simulink library "pwrsysTransf"  (R2016a)
settings: Solver=VariableStepAuto  SolverMode=SingleTasking  StartTime=0.0  StopTime=10.0  RelTol=1e-3
undefined symbols (not defined in the file or in its folder): fn
undefined symbols (not defined in the file): Ts_control
libraries: powerlib_meascontrol x32, pwrsysBasic x12, peTransforms x12, pwrsysTransf x12, pwrsysAMA x4, cstblocks x2
settings Model: Creator=daniemot  LastModifiedBy=ericfa
settings DebuggingCC: SFUnexpectedBacktrackingDiag=error  SFNoUnconditionalDefaultTransitionDiag=error
settings GRTTargetCC: TargetLangStandard=C99 (ISO)  GeneratePreprocessorConditionals=Use local settings
settings ConfigComp: CovMetricSettings=dwe  CovHtmlReporting=off  CovSaveCumulativeToWorkspaceVar=off  CovSaveSingleToWorkspaceVar=off  CovExternalEMLEnable=on

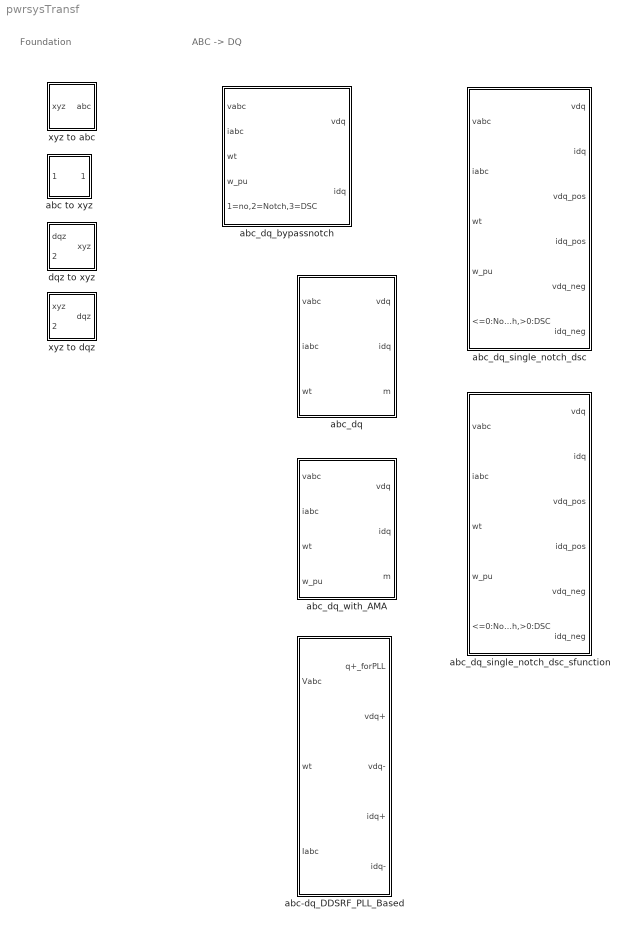
== system pwrsysTransf ==
  note: ABC -> DQ
  note: Foundation
  abc to xyz : Subsystem  mask(Clarke transformation){typeTransf=Amplitude-invariant}
      mask prompts: typeTransf "Type of transformation"
      mask init:
      | switch typeTransf
      |     case 1
      |         a = 1/3;
      |         b = 1/sqrt(3);
      |         c = sqrt(2)/3;
      |     case 2
      |         a = 1/sqrt(6);
      |         b = 1/sqrt(2);
      |         c = 1/sqrt(3);
      | end
      mask TypeOptions typeTransf: Amplitude-invariant | Power-invariant
  abc-dq_DDSRF_PLL_Based : Subsystem  mask(abc -> dq based on DDSRF PLL){Ts=Ts_control, fc=fn/2^0.5}
      mask prompts: Ts "Sampling time [s]"; fc "Cutout freq. low pass [Hz]"
      mask help:
      | abc -> dq transducer based on the Decoupled Double Synchronous Reference Frame PLL for Power Converters Control from Rodriguez 2007.
      | The PLL is not implemented, but an output with eq is available for using in a PLL
  abc_dq : Subsystem  mask(abc->dq with Matlab){Ts=0.001, fn=100, fcutoutv=1000, fcutouti=1000, zeta=0.707}
      mask prompts: Ts "Sampling time [s]"; fn "Notch frequency [Hz]"; fcutoutv "Cutout freq. low-pass for vdq meas. [Hz]"; fcutouti "Cutout freq. low-pass for idq meas. [Hz]"; zeta "Zeta for notch filters"
  abc_dq_bypassnotch : Subsystem  mask(abc->dq with Matlab){Ts=0.001, fn=100, fcutoutv=1000, fcutouti=1000, zeta=0.707}
      mask prompts: Ts "Sampling time [s]"; fn "Notch frequency [Hz]"; fcutoutv "Cutout freq. low-pass for vdq meas. [Hz]"; fcutouti "Cutout freq. low-pass for idq meas. [Hz]"; zeta "Zeta for notch filters"
      mask help:
      | To be done
      |
      | Max buffer size for DSC 500 samples
  abc_dq_single_notch_dsc : Subsystem  mask(abc->dq with Matlab){Ts=0.001, fn=100, zeta=0.707}
      mask prompts: Ts "Sampling time [s]"; fn "Notch frequency [Hz]"; zeta "Zeta for notch filters"
      mask help:
      | To be done
      |
      | Max buffer size for DSC 500 samples
  abc_dq_single_notch_dsc_sfunction : Subsystem  mask(abc->dq with Matlab){Ts=0.001, fn=100, zeta=0.707}
      mask prompts: Ts "Sampling time [s]"; fn "Notch frequency [Hz]"; zeta "Zeta for notch filters"
      mask help:
      | To be done
      |
      | Max buffer size for DSC 500 samples
  abc_dq_with_AMA : Subsystem  mask(abc->dq with Matlab){Ts=0.001, fn=100, fmin=0, fmax=0, fcutoutv=1000, fcutouti=1000}
      mask prompts: Ts "Sampling time [s]"; fn "Rated grid frequency [Hz]"; fmin "Min. acceptable grid freq [Hz]"; fmax "Max. acceptable grid freq [Hz]"; fcutoutv "Cutout freq. low-pass for vdq meas. [Hz]"; fcutouti "Cutout freq. low-pass for idq meas. [Hz]"
  dqz to xyz : Subsystem  mask(Inverse Park transformation){}
  xyz to abc : Subsystem  mask(Inverse Clarke transformation){typeTransf=Amplitude-invariant}
      mask prompts: typeTransf "Type of transformation"
      mask init:
      | switch typeTransf
      |     case 1
      |         a = 1;
      |         b = sqrt(3)/2;
      |         c = 1/2;
      |         d = 1/sqrt(2);
      |     case 2
      |         a = sqrt(2/3);
      |         b = 1/sqrt(2);
      |         c = 1/sqrt(6);
      |         d = 1/sqrt(3);
      | end
      mask TypeOptions typeTransf: Amplitude-invariant | Power-invariant
  xyz to dqz : Subsystem  mask(Inverse Park transformation){}

== system pwrsysTransf/abc to xyz ==
  note: Clark Transform
  abc : Inport
  Demux : Demux  Outputs=3
  Gain : Gain  Gain=c
  Gain1 : Gain  Gain=a
  Gain2 : Gain  Gain=b
  Gain4 : Gain  Gain=2
  Mux : Mux  Inputs=3
  Sum1 : Sum  Inputs=+-
  Sum2 : Sum  Inputs=+++
  Sum3 : Sum  Inputs=+--
  xyz : Outport
  wires:
  abc/1 -> Demux/1
  Demux/1 -> Sum2/1, Gain4/1  "a"
  Gain/1 -> Mux/3  "z"
  Gain2/1 -> Mux/2  "y"
  Gain1/1 -> Mux/1  "x"
  Mux/1 -> xyz/1
  Gain4/1 -> Sum3/1
  Demux/2 -> Sum2/2, Sum1/1, Sum3/2  "b"
  Demux/3 -> Sum2/3, Sum1/2, Sum3/3  "c"
  Sum3/1 -> Gain1/1  "B"
  Sum1/1 -> Gain2/1
  Sum2/1 -> Gain/1

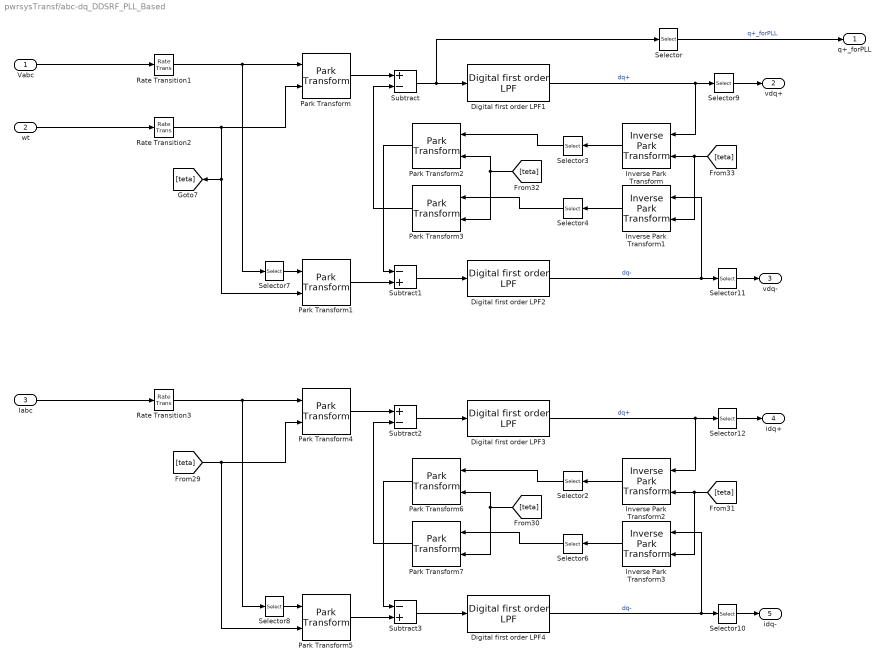
== system pwrsysTransf/abc-dq_DDSRF_PLL_Based ==
  Vabc : Inport
  wt : Inport  Port=2
  Iabc : Inport  Port=3
  Digital first order LPF{1..4} (4 alike) : pwrsysBasic/Digital first order LPF  Ts=Ts  fcutout=fc
  Inverse Park Transform{,1..3} (4 alike) : peTransforms/Inverse Park Transform  AxisAlignment=Q-axis  PowerInvariant=off
  Park Transform{,1..7} (8 alike) : peTransforms/Park Transform  AxisAlignment=Q-axis  PowerInvariant=off
  Rate Transition1 : RateTransition  OutPortSampleTime=Ts
  Rate Transition2 : RateTransition  OutPortSampleTime=Ts
  Rate Transition3 : RateTransition  OutPortSampleTime=Ts
  Selector : Selector  InputPortWidth=3  IndexOptions=Index vector (dialog)  Indices=2  OutputSizes=1
  Selector{9..12} (4 alike) : Selector  InputPortWidth=3  IndexOptions=Index vector (dialog)  Indices=[1 2]  OutputSizes=1
  Selector{2..4,6..8} (6 alike) : Selector  InputPortWidth=3  IndexOptions=Index vector (dialog)  Indices=[1 3 2]  OutputSizes=1
  Subtract : Sum  Inputs=+-
  Subtract1 : Sum  Inputs=-+
  Subtract2 : Sum  Inputs=+-
  Subtract3 : Sum  Inputs=-+
  q+_forPLL : Outport
  vdq+ : Outport  Port=2
  vdq- : Outport  Port=3
  idq+ : Outport  Port=4
  idq- : Outport  Port=5
  wires:
  Selector/1 -> q+_forPLL/1  "q+_forPLL"
  [teta] -> Inverse Park Transform2/2, Inverse Park Transform3/2
  Rate Transition3/1 -> Selector8/1, Park Transform4/1
  Selector11/1 -> vdq-/1
  Rate Transition1/1 -> Selector7/1, Park Transform/1
  Digital first order LPF4/1 -> Inverse Park Transform3/1, Selector10/1  "dq-"
  Inverse Park Transform3/1 -> Selector6/1
  Rate Transition2/1 -> [teta], Park Transform1/2, Park Transform/2
  Selector4/1 -> Park Transform3/1
  Iabc/1 -> Rate Transition3/1
  [teta] -> Park Transform6/2, Park Transform7/2
  Subtract2/1 -> Digital first order LPF3/1
  Park Transform1/1 -> Subtract1/2
  Selector6/1 -> Park Transform7/1
  Selector8/1 -> Park Transform5/1
  Park Transform7/1 -> Subtract2/2
  Digital first order LPF2/1 -> Selector11/1, Inverse Park Transform1/1  "dq-"
  Selector9/1 -> vdq+/1
  Inverse Park Transform1/1 -> Selector4/1
  Inverse Park Transform2/1 -> Selector2/1
  [teta] -> Park Transform2/2, Park Transform3/2
  Selector10/1 -> idq-/1
  Park Transform2/1 -> Subtract1/1
  Selector2/1 -> Park Transform6/1
  Park Transform5/1 -> Subtract3/2
  Subtract3/1 -> Digital first order LPF4/1
  Subtract1/1 -> Digital first order LPF2/1
  Park Transform/1 -> Subtract/1
  Digital first order LPF3/1 -> Inverse Park Transform2/1, Selector12/1  "dq+"
  Selector12/1 -> idq+/1
  Selector3/1 -> Park Transform2/1
  wt/1 -> Rate Transition2/1
  Park Transform6/1 -> Subtract3/1
  [teta] -> Park Transform5/2, Park Transform4/2
  Park Transform4/1 -> Subtract2/1
  Subtract/1 -> Digital first order LPF1/1, Selector/1
  [teta] -> Inverse Park Transform/2, Inverse Park Transform1/2
  Digital first order LPF1/1 -> Selector9/1, Inverse Park Transform/1  "dq+"
  Vabc/1 -> Rate Transition1/1
  Selector7/1 -> Park Transform1/1
  Inverse Park Transform/1 -> Selector3/1
  Park Transform3/1 -> Subtract/2

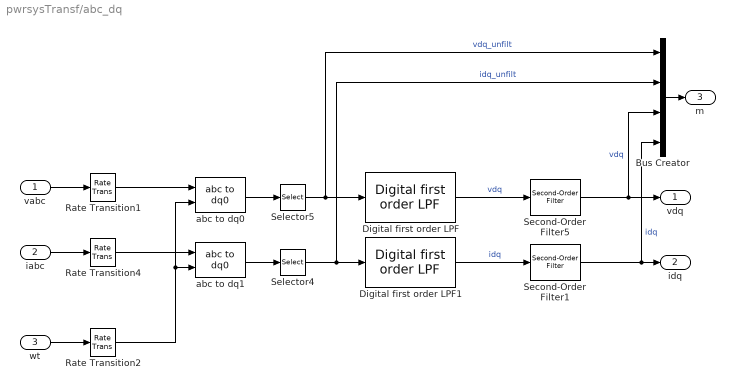
== system pwrsysTransf/abc_dq ==
  vabc : Inport
  iabc : Inport  Port=2
  wt : Inport  Port=3
  Bus Creator : BusCreator  Inputs=4
  Digital first order LPF : pwrsysBasic/Digital first order LPF  Ts=Ts  fcutout=fcutoutv
  Digital first order LPF1 : pwrsysBasic/Digital first order LPF  Ts=Ts  fcutout=fcutouti
  Rate Transition1 : RateTransition  OutPortSampleTime=Ts
  Rate Transition2 : RateTransition  OutPortSampleTime=Ts
  Rate Transition4 : RateTransition  OutPortSampleTime=Ts
  Second-Order Filter1 : powerlib_meascontrol/Filters/Second-Order Filter  FilterType=Bandstop (Notch)  Fo=fn  Zeta=zeta  Ts=Ts  Initialize=off  Vac_Init="[0,  0,  60]"  Vdc_Init=0  PlotResponse=off  FreqRange=[0, 1000, 0.1]
  Second-Order Filter5 : powerlib_meascontrol/Filters/Second-Order Filter  FilterType=Bandstop (Notch)  Fo=fn  Zeta=zeta  Ts=Ts  Initialize=off  Vac_Init="[0,  0,  60]"  Vdc_Init=0  PlotResponse=off  FreqRange=[0, 1000, 0.1]
  Selector4 : Selector  InputPortWidth=3  IndexOptions=Index vector (dialog)  Indices=[1 2]  OutputSizes=1
  Selector5 : Selector  InputPortWidth=3  IndexOptions=Index vector (dialog)  Indices=[1 2]  OutputSizes=1
  abc to dq0 : powerlib_meascontrol/Transformations/abc to dq0  Alignment=90 degrees behind phase A axis
  abc to dq1 : powerlib_meascontrol/Transformations/abc to dq0  Alignment=90 degrees behind phase A axis
  vdq : Outport
  idq : Outport  Port=2
  m : Outport  Port=3
  wires:
  abc to dq1/1 -> Selector4/1
  Selector5/1 -> Digital first order LPF/1, Bus Creator/1  "vdq_unfilt"
  Rate Transition1/1 -> abc to dq0/1
  Rate Transition2/1 -> abc to dq1/2, abc to dq0/2
  Selector4/1 -> Bus Creator/2, Digital first order LPF1/1  "idq_unfilt"
  Rate Transition4/1 -> abc to dq1/1
  abc to dq0/1 -> Selector5/1
  Bus Creator/1 -> m/1
  Second-Order Filter5/1 -> vdq/1, Bus Creator/3  "vdq"
  wt/1 -> Rate Transition2/1
  vabc/1 -> Rate Transition1/1
  iabc/1 -> Rate Transition4/1
  Digital first order LPF1/1 -> Second-Order Filter1/1  "idq"
  Digital first order LPF/1 -> Second-Order Filter5/1  "vdq"
  Second-Order Filter1/1 -> Bus Creator/4, idq/1  "idq"

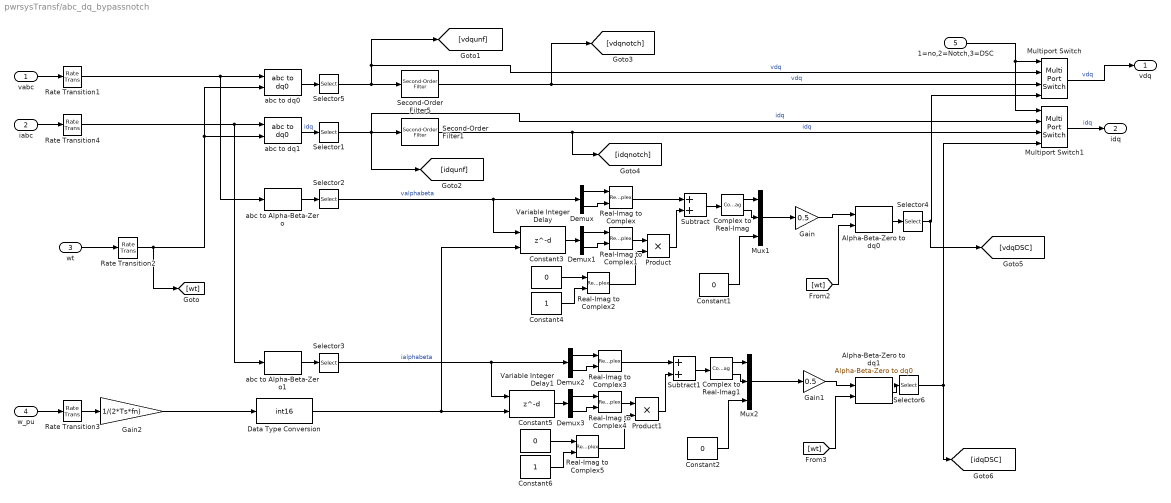
== system pwrsysTransf/abc_dq_bypassnotch ==
  vabc : Inport
  iabc : Inport  Port=2
  wt : Inport  Port=3
  w_pu : Inport  Port=4
  1=no,2=Notch,3=DSC : Inport  Port=5
  Alpha-Beta-Zero to dq0 : powerlib_meascontrol/Transformations/Alpha-Beta-Zero to dq0  Alignment=90 degrees behind phase A axis
  Alpha-Beta-Zero to dq1 : powerlib_meascontrol/Transformations/Alpha-Beta-Zero to dq0  Alignment=90 degrees behind phase A axis
  Complex to Real-Imag : ComplexToRealImag
  Complex to Real-Imag1 : ComplexToRealImag
  Constant{1..3,5} (4 alike) : Constant  Value=0
  Constant4 : Constant
  Constant6 : Constant
  Data Type Conversion : DataTypeConversion  OutDataTypeStr=int16  RndMeth=Round  SaturateOnIntegerOverflow=on
  Demux{,1..3} (4 alike) : Demux  Outputs=2
  Gain : Gain  Gain=0.5
  Gain1 : Gain  Gain=0.5
  Gain2 : Gain  Gain=1/(2*Ts*fn)
  Multiport Switch : MultiPortSwitch
  Multiport Switch1 : MultiPortSwitch
  Mux1 : Mux  Inputs=[1 1 1]
  Mux2 : Mux  Inputs=[1 1 1]
  Product : Product
  Product1 : Product
  Rate Transition1 : RateTransition  OutPortSampleTime=Ts
  Rate Transition2 : RateTransition  OutPortSampleTime=Ts
  Rate Transition3 : RateTransition  X0=1  OutPortSampleTime=Ts
  Rate Transition4 : RateTransition  OutPortSampleTime=Ts
  Real-Imag to Complex{,1..5} (6 alike) : RealImagToComplex
  Second-Order Filter1 : powerlib_meascontrol/Filters/Second-Order Filter  FilterType=Bandstop (Notch)  Fo=fn  Zeta=zeta  Ts=Ts  Initialize=off  Vac_Init="[0,  0,  60]"  Vdc_Init=0  PlotResponse=off  FreqRange=[0, 1000, 0.1]
  Second-Order Filter5 : powerlib_meascontrol/Filters/Second-Order Filter  FilterType=Bandstop (Notch)  Fo=fn  Zeta=zeta  Ts=Ts  Initialize=off  Vac_Init="[0,  0,  60]"  Vdc_Init=0  PlotResponse=off  FreqRange=[0, 1000, 0.1]
  Selector{1..6} (6 alike) : Selector  InputPortWidth=3  IndexOptions=Index vector (dialog)  Indices=[1 2]  OutputSizes=1
  Subtract : Sum
  Subtract1 : Sum
  Variable Integer Delay : Delay  DelayLengthSource=Input port  DelayLength=200  DelayLengthUpperLimit=500  SampleTime=Ts
      settings: InputPortMap=u0,p1
  Variable Integer Delay1 : Delay  DelayLengthSource=Input port  DelayLength=200  DelayLengthUpperLimit=500  SampleTime=Ts
      settings: InputPortMap=u0,p1
  abc to Alpha-Beta-Zero : powerlib_meascontrol/Transformations/abc to Alpha-Beta-Zero
  abc to Alpha-Beta-Zero1 : powerlib_meascontrol/Transformations/abc to Alpha-Beta-Zero
  abc to dq0 : powerlib_meascontrol/Transformations/abc to dq0  Alignment=90 degrees behind phase A axis
  abc to dq1 : powerlib_meascontrol/Transformations/abc to dq0  Alignment=90 degrees behind phase A axis
  vdq : Outport
  idq : Outport  Port=2
  wires:
  Rate Transition2/1 -> [wt], abc to dq1/2, abc to dq0/2
  wt/1 -> Rate Transition2/1
  abc to dq1/1 -> Selector1/1  "idq"
  Selector5/1 -> Second-Order Filter5/1, [vdqunf], Multiport Switch/2  "vdq"
  Second-Order Filter5/1 -> [vdqnotch], Multiport Switch/3  "vdq"
  Second-Order Filter1/1 -> [idqnotch], Multiport Switch1/3  "idq"
  abc to dq0/1 -> Selector5/1
  Selector1/1 -> [idqunf], Second-Order Filter1/1, Multiport Switch1/2  "idq"
  abc to Alpha-Beta-Zero/1 -> Selector2/1
  abc to Alpha-Beta-Zero1/1 -> Selector3/1
  Gain2/1 -> Data Type Conversion/1
  [wt] -> Alpha-Beta-Zero to dq0/2
  Alpha-Beta-Zero to dq0/1 -> Selector4/1
  Selector4/1 -> [vdqDSC], Multiport Switch/4
  Selector6/1 -> [idqDSC], Multiport Switch1/4
  [wt] -> Alpha-Beta-Zero to dq1/2
  Selector3/1 -> Demux2/1, Variable Integer Delay1/1  "ialphabeta"
  Alpha-Beta-Zero to dq1/1 -> Selector6/1
  Gain/1 -> Alpha-Beta-Zero to dq0/1
  Gain1/1 -> Alpha-Beta-Zero to dq1/1
  Variable Integer Delay/1 -> Demux1/1
  Constant1/1 -> Mux1/3
  Complex to Real-Imag/2 -> Mux1/2
  Constant4/1 -> Real-Imag to Complex2/2
  Complex to Real-Imag/1 -> Mux1/1
  Subtract/1 -> Complex to Real-Imag/1
  Real-Imag to Complex/1 -> Subtract/1
  Demux1/2 -> Real-Imag to Complex1/2
  Real-Imag to Complex1/1 -> Product/1
  Product/1 -> Subtract/2
  Real-Imag to Complex2/1 -> Product/2
  Constant3/1 -> Real-Imag to Complex2/1
  Demux1/1 -> Real-Imag to Complex1/1
  Demux/2 -> Real-Imag to Complex/2
  Demux/1 -> Real-Imag to Complex/1
  Selector2/1 -> Demux/1, Variable Integer Delay/1  "valphabeta"
  Mux1/1 -> Gain/1
  Mux2/1 -> Gain1/1
  Demux2/1 -> Real-Imag to Complex3/1
  Constant5/1 -> Real-Imag to Complex5/1
  Real-Imag to Complex5/1 -> Product1/2
  Demux3/1 -> Real-Imag to Complex4/1
  Product1/1 -> Subtract1/2
  Demux2/2 -> Real-Imag to Complex3/2
  Demux3/2 -> Real-Imag to Complex4/2
  Real-Imag to Complex3/1 -> Subtract1/1
  Constant6/1 -> Real-Imag to Complex5/2
  Real-Imag to Complex4/1 -> Product1/1
  Complex to Real-Imag1/1 -> Mux2/1
  Constant2/1 -> Mux2/3
  Complex to Real-Imag1/2 -> Mux2/2
  Variable Integer Delay1/1 -> Demux3/1
  Subtract1/1 -> Complex to Real-Imag1/1
  Rate Transition1/1 -> abc to Alpha-Beta-Zero/1, abc to dq0/1
  Rate Transition4/1 -> abc to Alpha-Beta-Zero1/1, abc to dq1/1
  w_pu/1 -> Rate Transition3/1
  Rate Transition3/1 -> Gain2/1
  vabc/1 -> Rate Transition1/1
  iabc/1 -> Rate Transition4/1
  Data Type Conversion/1 -> Variable Integer Delay1/2, Variable Integer Delay/2
  Multiport Switch/1 -> vdq/1  "vdq"
  Multiport Switch1/1 -> idq/1  "idq"
  1=no,2=Notch,3=DSC/1 -> Multiport Switch1/1, Multiport Switch/1

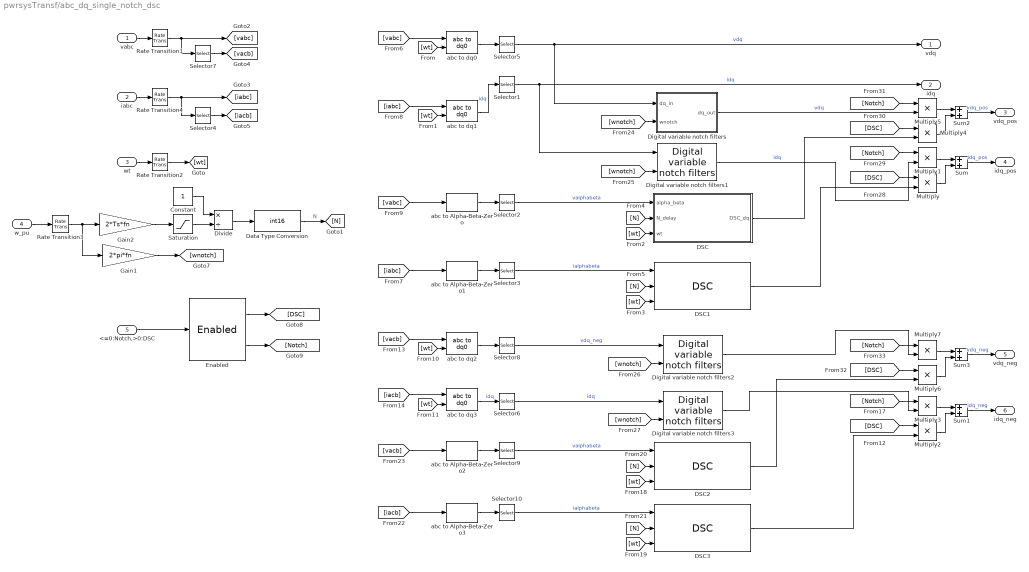
== system pwrsysTransf/abc_dq_single_notch_dsc ==
  vabc : Inport
  iabc : Inport  Port=2
  wt : Inport  Port=3
  w_pu : Inport  Port=4
  <=0:Notch,>0:DSC : Inport  Port=5
  Constant : Constant
  DSC : Subsystem
  DSC1 : pwrsysTransf/abc_dq_single_notch_dsc/DSC
  DSC2 : pwrsysTransf/abc_dq_single_notch_dsc/DSC
  DSC3 : pwrsysTransf/abc_dq_single_notch_dsc/DSC
  Data Type Conversion : DataTypeConversion  OutDataTypeStr=int16  RndMeth=Round  SaturateOnIntegerOverflow=on
  Digital variable notch filters : Subsystem
  Digital variable notch filters1 : pwrsysTransf/abc_dq_single_notch_dsc/Digital variable notch filters
  Digital variable notch filters2 : pwrsysTransf/abc_dq_single_notch_dsc/Digital variable notch filters
  Digital variable notch filters3 : pwrsysTransf/abc_dq_single_notch_dsc/Digital variable notch filters
  Divide : Product  Inputs=*/
  Enabled : pwrsysBasic/Enabled
  Gain1 : Gain  Gain=2*pi*fn
  Gain2 : Gain  Gain=2*Ts*fn
  Multiply{,1..7} (8 alike) : Product
  Rate Transition1 : RateTransition  OutPortSampleTime=Ts
  Rate Transition2 : RateTransition  OutPortSampleTime=Ts
  Rate Transition3 : RateTransition  X0=1  OutPortSampleTime=Ts
  Rate Transition4 : RateTransition  OutPortSampleTime=Ts
  Saturation : Saturate  UpperLimit=inf  LowerLimit=0.000001
  Selector{1..3,5..6,8..10} (8 alike) : Selector  InputPortWidth=3  IndexOptions=Index vector (dialog)  Indices=[1 2]  OutputSizes=1
  Selector4 : Selector  InputPortWidth=3  IndexOptions=Index vector (dialog)  Indices=[1 3 2]  OutputSizes=1
  Selector7 : Selector  InputPortWidth=3  IndexOptions=Index vector (dialog)  Indices=[1 3 2]  OutputSizes=1
  Sum{,1..3} (4 alike) : Sum
  abc to Alpha-Beta-Zero{,1..3} (4 alike) : powerlib_meascontrol/Transformations/abc to Alpha-Beta-Zero
  abc to dq{0..3} (4 alike) : powerlib_meascontrol/Transformations/abc to dq0  Alignment=90 degrees behind phase A axis
  vdq : Outport
  idq : Outport  Port=2
  vdq_pos : Outport  Port=3
  idq_pos : Outport  Port=4
  vdq_neg : Outport  Port=5
  idq_neg : Outport  Port=6
  wires:
  wt/1 -> Rate Transition2/1
  abc to dq1/1 -> Selector1/1  "idq"
  Selector5/1 -> Digital variable notch filters/1(dq_in), vdq/1  "vdq"
  abc to dq0/1 -> Selector5/1
  Selector1/1 -> Digital variable notch filters1/1, idq/1  "idq"
  abc to Alpha-Beta-Zero/1 -> Selector2/1
  abc to Alpha-Beta-Zero1/1 -> Selector3/1
  DSC/1(DSC_dq) -> Multiply4/2
  Selector3/1 -> DSC1/1  "ialphabeta"
  [vabc] -> abc to dq0/1
  [iabc] -> abc to dq1/1
  vabc/1 -> Rate Transition1/1
  iabc/1 -> Rate Transition4/1
  Selector2/1 -> DSC/1(alpha_beta)  "valphabeta"
  Digital variable notch filters/1(dq_out) -> Multiply5/2  "vdq"
  Digital variable notch filters1/1 -> Multiply1/2  "idq"
  DSC1/1 -> Multiply/2
  Sum2/1 -> vdq_pos/1  "vdq_pos"
  Sum/1 -> idq_pos/1  "idq_pos"
  Rate Transition2/1 -> [wt]
  [wt] -> abc to dq0/2
  [wt] -> abc to dq1/2
  [wt] -> DSC/3(wt)
  [wt] -> DSC1/3
  [N] -> DSC/2(N_delay)
  [N] -> DSC1/2
  Data Type Conversion/1 -> [N]  "N"
  Rate Transition1/1 -> Selector7/1, [vabc]
  Selector7/1 -> [vacb]
  Rate Transition4/1 -> Selector4/1, [iabc]
  Selector4/1 -> [iacb]
  [vabc] -> abc to Alpha-Beta-Zero/1
  [iabc] -> abc to Alpha-Beta-Zero1/1
  [wt] -> abc to dq3/2
  abc to dq2/1 -> Selector8/1
  Selector8/1 -> Digital variable notch filters2/1  "vdq_neg"
  [vacb] -> abc to dq2/1
  [wt] -> abc to dq2/2
  abc to dq3/1 -> Selector6/1  "idq"
  [iacb] -> abc to dq3/1
  Sum3/1 -> vdq_neg/1  "vdq_neg"
  Sum1/1 -> idq_neg/1  "idq_neg"
  Digital variable notch filters2/1 -> Multiply7/2
  Selector6/1 -> Digital variable notch filters3/1  "idq"
  Digital variable notch filters3/1 -> Multiply3/2
  abc to Alpha-Beta-Zero3/1 -> Selector10/1
  Selector10/1 -> DSC3/1  "ialphabeta"
  abc to Alpha-Beta-Zero2/1 -> Selector9/1
  [iacb] -> abc to Alpha-Beta-Zero3/1
  [wt] -> DSC2/3
  [vacb] -> abc to Alpha-Beta-Zero2/1
  DSC2/1 -> Multiply6/2
  Selector9/1 -> DSC2/1  "valphabeta"
  [N] -> DSC3/2
  [N] -> DSC2/2
  DSC3/1 -> Multiply2/2
  [wt] -> DSC3/3
  Gain2/1 -> Saturation/1
  Saturation/1 -> Divide/2
  Constant/1 -> Divide/1
  Rate Transition3/1 -> Gain1/1, Gain2/1
  Divide/1 -> Data Type Conversion/1
  w_pu/1 -> Rate Transition3/1
  Gain1/1 -> [wnotch]
  [wnotch] -> Digital variable notch filters/2(wnotch)
  [wnotch] -> Digital variable notch filters1/2
  [wnotch] -> Digital variable notch filters2/2
  [wnotch] -> Digital variable notch filters3/2
  <=0:Notch,>0:DSC/1 -> Enabled/1
  Enabled/1 -> [DSC]
  Enabled/2 -> [Notch]
  [DSC] -> Multiply/1
  [Notch] -> Multiply1/1
  Multiply1/1 -> Sum/1
  Multiply/1 -> Sum/2
  [Notch] -> Multiply3/1
  [DSC] -> Multiply2/1
  Multiply3/1 -> Sum1/1
  Multiply2/1 -> Sum1/2
  [Notch] -> Multiply5/1
  Multiply4/1 -> Sum2/2
  [DSC] -> Multiply4/1
  Multiply5/1 -> Sum2/1
  [Notch] -> Multiply7/1
  Multiply6/1 -> Sum3/2
  [DSC] -> Multiply6/1
  Multiply7/1 -> Sum3/1

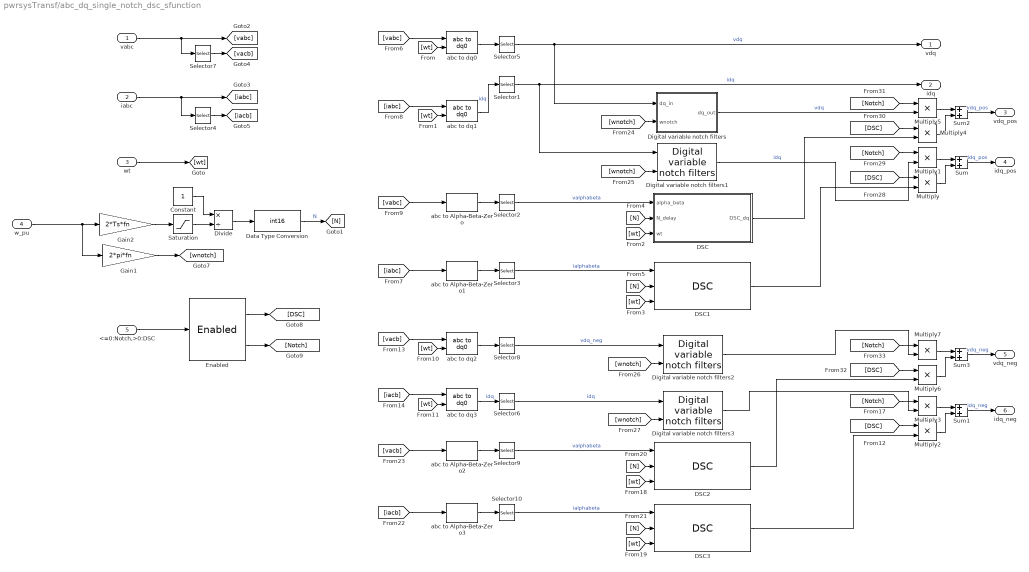
== system pwrsysTransf/abc_dq_single_notch_dsc_sfunction ==
  vabc : Inport
  iabc : Inport  Port=2
  wt : Inport  Port=3
  w_pu : Inport  Port=4
  <=0:Notch,>0:DSC : Inport  Port=5
  Constant : Constant
  DSC : Subsystem
  DSC1 : pwrsysTransf/abc_dq_single_notch_dsc/DSC
  DSC2 : pwrsysTransf/abc_dq_single_notch_dsc/DSC
  DSC3 : pwrsysTransf/abc_dq_single_notch_dsc/DSC
  Data Type Conversion : DataTypeConversion  OutDataTypeStr=int16  RndMeth=Round  SaturateOnIntegerOverflow=on
  Digital variable notch filters : Subsystem
  Digital variable notch filters1 : pwrsysTransf/abc_dq_single_notch_dsc_sfunction/Digital variable notch filters
  Digital variable notch filters2 : pwrsysTransf/abc_dq_single_notch_dsc_sfunction/Digital variable notch filters
  Digital variable notch filters3 : pwrsysTransf/abc_dq_single_notch_dsc_sfunction/Digital variable notch filters
  Divide : Product  Inputs=*/
  Enabled : pwrsysBasic/Enabled
  Gain1 : Gain  Gain=2*pi*fn
  Gain2 : Gain  Gain=2*Ts*fn
  Multiply{,1..7} (8 alike) : Product
  Saturation : Saturate  UpperLimit=inf  LowerLimit=0.000001
  Selector{1..3,5..6,8..10} (8 alike) : Selector  InputPortWidth=3  IndexOptions=Index vector (dialog)  Indices=[1 2]  OutputSizes=1
  Selector4 : Selector  InputPortWidth=3  IndexOptions=Index vector (dialog)  Indices=[1 3 2]  OutputSizes=1
  Selector7 : Selector  InputPortWidth=3  IndexOptions=Index vector (dialog)  Indices=[1 3 2]  OutputSizes=1
  Sum{,1..3} (4 alike) : Sum
  abc to Alpha-Beta-Zero{,1..3} (4 alike) : powerlib_meascontrol/Transformations/abc to Alpha-Beta-Zero
  abc to dq{0..3} (4 alike) : powerlib_meascontrol/Transformations/abc to dq0  Alignment=90 degrees behind phase A axis
  vdq : Outport
  idq : Outport  Port=2
  vdq_pos : Outport  Port=3
  idq_pos : Outport  Port=4
  vdq_neg : Outport  Port=5
  idq_neg : Outport  Port=6
  wires:
  Multiply7/1 -> Sum3/1
  [DSC] -> Multiply6/1
  Multiply6/1 -> Sum3/2
  [Notch] -> Multiply7/1
  Multiply5/1 -> Sum2/1
  [DSC] -> Multiply4/1
  Multiply4/1 -> Sum2/2
  [Notch] -> Multiply5/1
  Multiply2/1 -> Sum1/2
  Multiply3/1 -> Sum1/1
  [DSC] -> Multiply2/1
  [Notch] -> Multiply3/1
  Multiply/1 -> Sum/2
  Multiply1/1 -> Sum/1
  [Notch] -> Multiply1/1
  [DSC] -> Multiply/1
  Enabled/2 -> [Notch]
  Enabled/1 -> [DSC]
  <=0:Notch,>0:DSC/1 -> Enabled/1
  [wnotch] -> Digital variable notch filters3/2
  [wnotch] -> Digital variable notch filters2/2
  [wnotch] -> Digital variable notch filters1/2
  [wnotch] -> Digital variable notch filters/2(wnotch)
  Gain1/1 -> [wnotch]
  Divide/1 -> Data Type Conversion/1
  w_pu/1 -> Gain2/1, Gain1/1
  Constant/1 -> Divide/1
  Saturation/1 -> Divide/2
  Gain2/1 -> Saturation/1
  [wt] -> DSC3/3
  DSC3/1 -> Multiply2/2
  [N] -> DSC2/2
  [N] -> DSC3/2
  Selector9/1 -> DSC2/1  "valphabeta"
  DSC2/1 -> Multiply6/2
  [vacb] -> abc to Alpha-Beta-Zero2/1
  [wt] -> DSC2/3
  [iacb] -> abc to Alpha-Beta-Zero3/1
  abc to Alpha-Beta-Zero2/1 -> Selector9/1
  Selector10/1 -> DSC3/1  "ialphabeta"
  abc to Alpha-Beta-Zero3/1 -> Selector10/1
  Digital variable notch filters3/1 -> Multiply3/2
  Selector6/1 -> Digital variable notch filters3/1  "idq"
  Digital variable notch filters2/1 -> Multiply7/2
  Sum1/1 -> idq_neg/1  "idq_neg"
  Sum3/1 -> vdq_neg/1  "vdq_neg"
  [iacb] -> abc to dq3/1
  abc to dq3/1 -> Selector6/1  "idq"
  [wt] -> abc to dq2/2
  [vacb] -> abc to dq2/1
  Selector8/1 -> Digital variable notch filters2/1  "vdq_neg"
  abc to dq2/1 -> Selector8/1
  [wt] -> abc to dq3/2
  [iabc] -> abc to Alpha-Beta-Zero1/1
  [vabc] -> abc to Alpha-Beta-Zero/1
  Selector4/1 -> [iacb]
  iabc/1 -> [iabc], Selector4/1
  Selector7/1 -> [vacb]
  vabc/1 -> [vabc], Selector7/1
  Data Type Conversion/1 -> [N]  "N"
  [N] -> DSC1/2
  [N] -> DSC/2(N_delay)
  [wt] -> DSC1/3
  [wt] -> DSC/3(wt)
  [wt] -> abc to dq1/2
  [wt] -> abc to dq0/2
  wt/1 -> [wt]
  Sum/1 -> idq_pos/1  "idq_pos"
  Sum2/1 -> vdq_pos/1  "vdq_pos"
  DSC1/1 -> Multiply/2
  Digital variable notch filters1/1 -> Multiply1/2  "idq"
  Digital variable notch filters/1(dq_out) -> Multiply5/2  "vdq"
  Selector2/1 -> DSC/1(alpha_beta)  "valphabeta"
  [iabc] -> abc to dq1/1
  [vabc] -> abc to dq0/1
  Selector3/1 -> DSC1/1  "ialphabeta"
  DSC/1(DSC_dq) -> Multiply4/2
  abc to Alpha-Beta-Zero1/1 -> Selector3/1
  abc to Alpha-Beta-Zero/1 -> Selector2/1
  Selector1/1 -> Digital variable notch filters1/1, idq/1  "idq"
  abc to dq0/1 -> Selector5/1
  Selector5/1 -> vdq/1, Digital variable notch filters/1(dq_in)  "vdq"
  abc to dq1/1 -> Selector1/1  "idq"

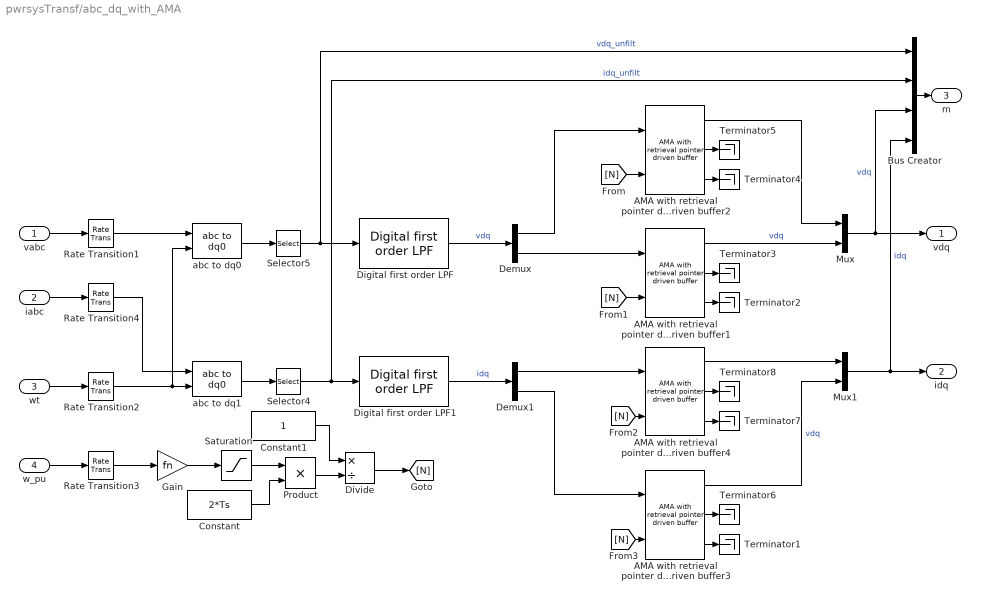
== system pwrsysTransf/abc_dq_with_AMA ==
  vabc : Inport
  iabc : Inport  Port=2
  wt : Inport  Port=3
  w_pu : Inport  Port=4
  AMA with retrieval pointer driven buffer{1..4} (4 alike) : pwrsysAMA/AMA with retrieval pointer driven buffer  NbSize=1/(2*fmin*Ts)  Ts=Ts
  Bus Creator : BusCreator  Inputs=4
  Constant : Constant  Value=2*Ts
  Constant1 : Constant
  Demux : Demux  Outputs=2
  Demux1 : Demux  Outputs=2
  Digital first order LPF : pwrsysBasic/Digital first order LPF  Ts=Ts  fcutout=fcutoutv
  Digital first order LPF1 : pwrsysBasic/Digital first order LPF  Ts=Ts  fcutout=fcutouti
  Divide : Product  Inputs=*/
  Gain : Gain  Gain=fn
  Mux : Mux  Inputs=2
  Mux1 : Mux  Inputs=2
  Product : Product
  Rate Transition1 : RateTransition  OutPortSampleTime=Ts
  Rate Transition2 : RateTransition  OutPortSampleTime=Ts
  Rate Transition3 : RateTransition  X0=1  OutPortSampleTime=Ts
  Rate Transition4 : RateTransition  OutPortSampleTime=Ts
  Saturation : Saturate  UpperLimit=fmax  LowerLimit=fmin
  Selector4 : Selector  InputPortWidth=3  IndexOptions=Index vector (dialog)  Indices=[1 2]  OutputSizes=1
  Selector5 : Selector  InputPortWidth=3  IndexOptions=Index vector (dialog)  Indices=[1 2]  OutputSizes=1
  Terminator{1..8} (8 alike) : Terminator
  abc to dq0 : powerlib_meascontrol/Transformations/abc to dq0  Alignment=90 degrees behind phase A axis
  abc to dq1 : powerlib_meascontrol/Transformations/abc to dq0  Alignment=90 degrees behind phase A axis
  vdq : Outport
  idq : Outport  Port=2
  m : Outport  Port=3
  wires:
  Digital first order LPF/1 -> Demux/1  "vdq"
  abc to dq1/1 -> Selector4/1
  Mux1/1 -> Bus Creator/4, idq/1  "idq"
  Selector5/1 -> Digital first order LPF/1, Bus Creator/1  "vdq_unfilt"
  Rate Transition1/1 -> abc to dq0/1
  Rate Transition2/1 -> abc to dq0/2, abc to dq1/2
  Selector4/1 -> Bus Creator/2, Digital first order LPF1/1  "idq_unfilt"
  Rate Transition4/1 -> abc to dq1/1
  abc to dq0/1 -> Selector5/1
  Bus Creator/1 -> m/1
  Mux/1 -> Bus Creator/3, vdq/1  "vdq"
  wt/1 -> Rate Transition2/1
  vabc/1 -> Rate Transition1/1
  iabc/1 -> Rate Transition4/1
  AMA with retrieval pointer driven buffer1/3 -> Terminator2/1
  AMA with retrieval pointer driven buffer1/2 -> Terminator3/1
  w_pu/1 -> Rate Transition3/1
  Rate Transition3/1 -> Gain/1
  Gain/1 -> Saturation/1
  Saturation/1 -> Product/1
  Constant/1 -> Product/2
  Product/1 -> Divide/2
  Constant1/1 -> Divide/1
  Divide/1 -> [N]
  Demux/1 -> AMA with retrieval pointer driven buffer2/1
  Demux/2 -> AMA with retrieval pointer driven buffer1/1
  AMA with retrieval pointer driven buffer2/3 -> Terminator4/1
  AMA with retrieval pointer driven buffer2/2 -> Terminator5/1
  AMA with retrieval pointer driven buffer2/1 -> Mux/1
  AMA with retrieval pointer driven buffer1/1 -> Mux/2  "vdq"
  AMA with retrieval pointer driven buffer3/1 -> Mux1/2  "vdq"
  AMA with retrieval pointer driven buffer4/2 -> Terminator8/1
  Demux1/1 -> AMA with retrieval pointer driven buffer4/1
  Demux1/2 -> AMA with retrieval pointer driven buffer3/1
  AMA with retrieval pointer driven buffer4/3 -> Terminator7/1
  AMA with retrieval pointer driven buffer3/3 -> Terminator1/1
  AMA with retrieval pointer driven buffer4/1 -> Mux1/1
  AMA with retrieval pointer driven buffer3/2 -> Terminator6/1
  Digital first order LPF1/1 -> Demux1/1  "idq"
  [N] -> AMA with retrieval pointer driven buffer2/2
  [N] -> AMA with retrieval pointer driven buffer1/2
  [N] -> AMA with retrieval pointer driven buffer4/2
  [N] -> AMA with retrieval pointer driven buffer3/2

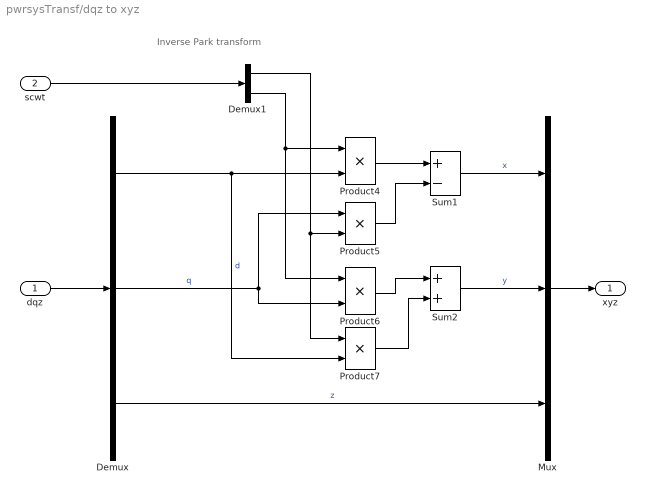
== system pwrsysTransf/dqz to xyz ==
  note: Inverse Park transform
  dqz : Inport
  scwt : Inport  Port=2
  Demux : Demux  Outputs=3
  Demux1 : Demux  Outputs=2
  Mux : Mux  Inputs=3
  Product{4..7} (4 alike) : Product
  Sum1 : Sum  Inputs=+-
  Sum2 : Sum
  xyz : Outport
  wires:
  dqz/1 -> Demux/1
  Demux/1 -> Product7/2, Product4/2  "d"
  Demux1/2 -> Product4/1, Product6/1
  Product5/1 -> Sum1/2
  Product4/1 -> Sum1/1
  Demux1/1 -> Product7/1, Product5/2
  Demux/2 -> Product6/2, Product5/1  "q"
  scwt/1 -> Demux1/1
  Product6/1 -> Sum2/1
  Product7/1 -> Sum2/2
  Mux/1 -> xyz/1
  Demux/3 -> Mux/3  "z"
  Sum2/1 -> Mux/2  "y"
  Sum1/1 -> Mux/1  "x"

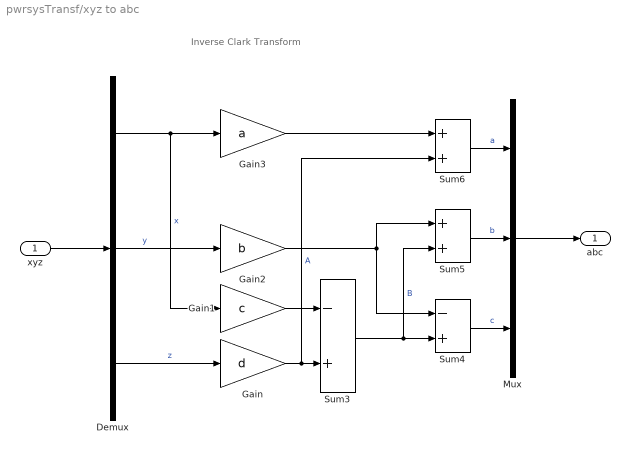
== system pwrsysTransf/xyz to abc ==
  note: Inverse Clark Transform
  xyz : Inport
  Demux : Demux  Outputs=3
  Gain : Gain  Gain=d
  Gain1 : Gain  Gain=c
  Gain2 : Gain  Gain=b
  Gain3 : Gain  Gain=a
  Mux : Mux  Inputs=3
  Sum3 : Sum  Inputs=-+
  Sum4 : Sum  Inputs=-+
  Sum5 : Sum
  Sum6 : Sum
  abc : Outport
  wires:
  xyz/1 -> Demux/1
  Demux/2 -> Gain2/1  "y"
  Demux/1 -> Gain3/1, Gain1/1  "x"
  Demux/3 -> Gain/1  "z"
  Gain1/1 -> Sum3/1
  Gain/1 -> Sum6/2, Sum3/2  "A"
  Gain2/1 -> Sum5/1, Sum4/1
  Sum3/1 -> Sum5/2, Sum4/2  "B"
  Sum4/1 -> Mux/3  "c"
  Sum5/1 -> Mux/2  "b"
  Sum6/1 -> Mux/1  "a"
  Gain3/1 -> Sum6/1
  Mux/1 -> abc/1

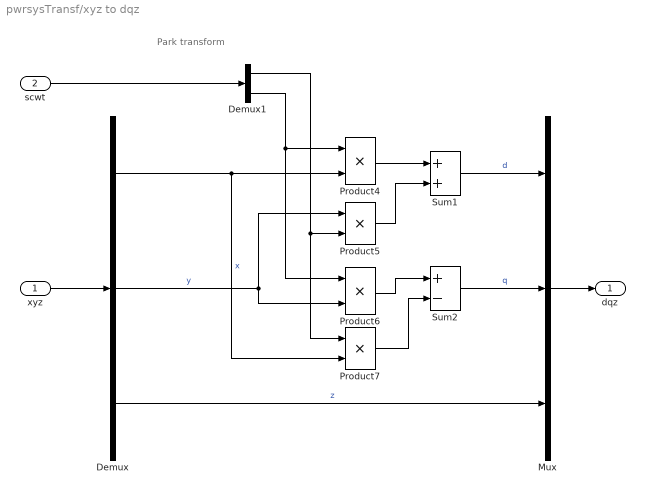
== system pwrsysTransf/xyz to dqz ==
  note: Park transform
  xyz : Inport
  scwt : Inport  Port=2
  Demux : Demux  Outputs=3
  Demux1 : Demux  Outputs=2
  Mux : Mux  Inputs=3
  Product{4..7} (4 alike) : Product
  Sum1 : Sum
  Sum2 : Sum  Inputs=+-
  dqz : Outport
  wires:
  Sum1/1 -> Mux/1  "d"
  Sum2/1 -> Mux/2  "q"
  Demux/3 -> Mux/3  "z"
  Mux/1 -> dqz/1
  Product7/1 -> Sum2/2
  Product6/1 -> Sum2/1
  scwt/1 -> Demux1/1
  Demux/2 -> Product5/1, Product6/2  "y"
  Demux1/1 -> Product5/2, Product7/1
  Product4/1 -> Sum1/1
  Product5/1 -> Sum1/2
  Demux1/2 -> Product6/1, Product4/1
  Demux/1 -> Product4/2, Product7/2  "x"
  xyz/1 -> Demux/1

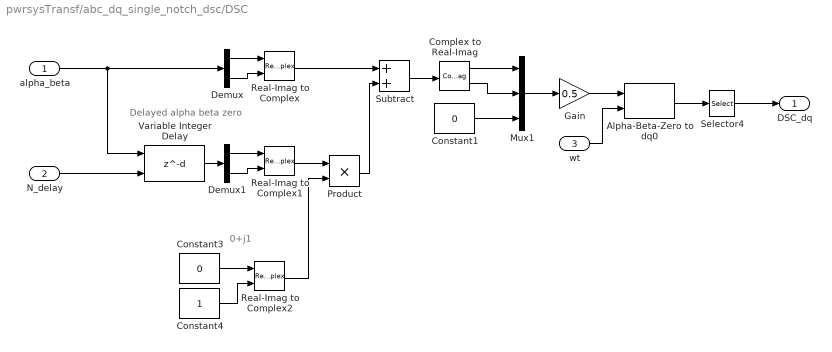
== system pwrsysTransf/abc_dq_single_notch_dsc/DSC ==
  note: 0+j1
  note: Delayed alpha beta zero
  alpha_beta : Inport
  N_delay : Inport  Port=2
  wt : Inport  Port=3
  Alpha-Beta-Zero to dq0 : powerlib_meascontrol/Transformations/Alpha-Beta-Zero to dq0  Alignment=90 degrees behind phase A axis
  Complex to Real-Imag : ComplexToRealImag
  Constant1 : Constant  Value=0
  Constant3 : Constant  Value=0
  Constant4 : Constant
  Demux : Demux  Outputs=2
  Demux1 : Demux  Outputs=2
  Gain : Gain  Gain=0.5
  Mux1 : Mux  Inputs=[1 1 1]
  Product : Product
  Real-Imag to Complex : RealImagToComplex
  Real-Imag to Complex1 : RealImagToComplex
  Real-Imag to Complex2 : RealImagToComplex
  Selector4 : Selector  InputPortWidth=3  IndexOptions=Index vector (dialog)  Indices=[1 2]  OutputSizes=1
  Subtract : Sum
  Variable Integer Delay : Delay  DelayLengthSource=Input port  DelayLength=200  DelayLengthUpperLimit=500  SampleTime=Ts
      settings: InputPortMap=u0,p1
  DSC_dq : Outport
  wires:
  Product/1 -> Subtract/2
  Demux/1 -> Real-Imag to Complex/1
  Real-Imag to Complex1/1 -> Product/1
  Demux1/1 -> Real-Imag to Complex1/1
  wt/1 -> Alpha-Beta-Zero to dq0/2
  Complex to Real-Imag/1 -> Mux1/1
  Variable Integer Delay/1 -> Demux1/1
  Demux1/2 -> Real-Imag to Complex1/2
  N_delay/1 -> Variable Integer Delay/2
  Gain/1 -> Alpha-Beta-Zero to dq0/1
  Constant3/1 -> Real-Imag to Complex2/1
  Real-Imag to Complex/1 -> Subtract/1
  alpha_beta/1 -> Variable Integer Delay/1, Demux/1
  Real-Imag to Complex2/1 -> Product/2
  Subtract/1 -> Complex to Real-Imag/1
  Constant1/1 -> Mux1/3
  Demux/2 -> Real-Imag to Complex/2
  Constant4/1 -> Real-Imag to Complex2/2
  Complex to Real-Imag/2 -> Mux1/2
  Mux1/1 -> Gain/1
  Alpha-Beta-Zero to dq0/1 -> Selector4/1
  Selector4/1 -> DSC_dq/1

== system pwrsysTransf/abc_dq_single_notch_dsc/Digital variable notch filters ==
  dq_in : Inport
  wnotch : Inport  Port=2
  Constant : Constant  Value=0
  Constant1 : Constant  Value=zeta
  Constant2 : Constant  Value=0
  Constant3 : Constant  Value=zeta
  Demux : Demux  Outputs=2
  Discrete Varying Notch1 : cstblocks/Linear Parameter Varying/Discrete Varying Notch  w0=0  Ts=Ts
  Discrete Varying Notch2 : cstblocks/Linear Parameter Varying/Discrete Varying Notch  w0=0  Ts=Ts
  Mux : Mux  Inputs=2
  dq_out : Outport
  wires:
  Demux/2 -> Discrete Varying Notch1/1
  dq_in/1 -> Demux/1
  Constant2/1 -> Discrete Varying Notch1/3
  wnotch/1 -> Discrete Varying Notch1/2, Discrete Varying Notch2/2
  Constant3/1 -> Discrete Varying Notch1/4
  Mux/1 -> dq_out/1
  Discrete Varying Notch1/1 -> Mux/2
  Demux/1 -> Discrete Varying Notch2/1
  Constant/1 -> Discrete Varying Notch2/3
  Constant1/1 -> Discrete Varying Notch2/4
  Discrete Varying Notch2/1 -> Mux/1

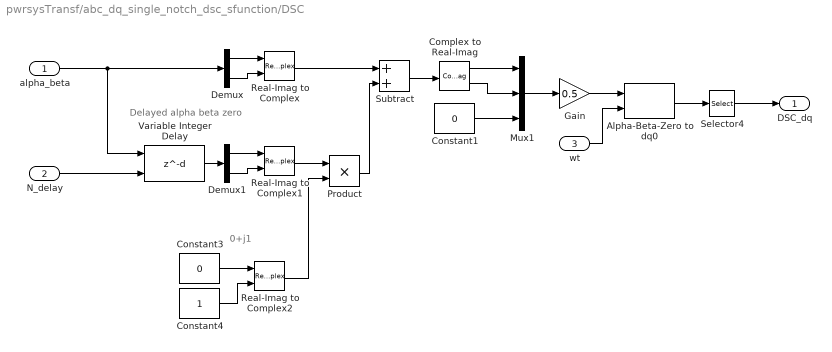
== system pwrsysTransf/abc_dq_single_notch_dsc_sfunction/DSC ==
  note: Delayed alpha beta zero
  note: 0+j1
  alpha_beta : Inport
  N_delay : Inport  Port=2
  wt : Inport  Port=3
  Alpha-Beta-Zero to dq0 : powerlib_meascontrol/Transformations/Alpha-Beta-Zero to dq0  Alignment=90 degrees behind phase A axis
  Complex to Real-Imag : ComplexToRealImag
  Constant1 : Constant  Value=0
  Constant3 : Constant  Value=0
  Constant4 : Constant
  Demux : Demux  Outputs=2
  Demux1 : Demux  Outputs=2
  Gain : Gain  Gain=0.5
  Mux1 : Mux  Inputs=[1 1 1]
  Product : Product
  Real-Imag to Complex : RealImagToComplex
  Real-Imag to Complex1 : RealImagToComplex
  Real-Imag to Complex2 : RealImagToComplex
  Selector4 : Selector  InputPortWidth=3  IndexOptions=Index vector (dialog)  Indices=[1 2]  OutputSizes=1
  Subtract : Sum
  Variable Integer Delay : Delay  DelayLengthSource=Input port  DelayLength=200  DelayLengthUpperLimit=500  SampleTime=Ts
      settings: InputPortMap=u0,p1
  DSC_dq : Outport
  wires:
  Selector4/1 -> DSC_dq/1
  Alpha-Beta-Zero to dq0/1 -> Selector4/1
  Mux1/1 -> Gain/1
  Complex to Real-Imag/2 -> Mux1/2
  Constant4/1 -> Real-Imag to Complex2/2
  Demux/2 -> Real-Imag to Complex/2
  Constant1/1 -> Mux1/3
  Subtract/1 -> Complex to Real-Imag/1
  Real-Imag to Complex2/1 -> Product/2
  alpha_beta/1 -> Demux/1, Variable Integer Delay/1
  Real-Imag to Complex/1 -> Subtract/1
  Constant3/1 -> Real-Imag to Complex2/1
  Gain/1 -> Alpha-Beta-Zero to dq0/1
  N_delay/1 -> Variable Integer Delay/2
  Demux1/2 -> Real-Imag to Complex1/2
  Variable Integer Delay/1 -> Demux1/1
  Complex to Real-Imag/1 -> Mux1/1
  wt/1 -> Alpha-Beta-Zero to dq0/2
  Demux1/1 -> Real-Imag to Complex1/1
  Real-Imag to Complex1/1 -> Product/1
  Demux/1 -> Real-Imag to Complex/1
  Product/1 -> Subtract/2

== system pwrsysTransf/abc_dq_single_notch_dsc_sfunction/Digital variable notch filters ==
  dq_in : Inport
  wnotch : Inport  Port=2
  Constant : Constant  Value=0
  Constant1 : Constant  Value=zeta
  Constant2 : Constant  Value=0
  Constant3 : Constant  Value=zeta
  Demux : Demux  Outputs=2
  Discrete Notch : pwrsysBasic/Discrete Notch  Ts=Ts
  Discrete Notch1 : pwrsysBasic/Discrete Notch  Ts=Ts
  Mux : Mux  Inputs=2
  dq_out : Outport
  wires:
  Discrete Notch/1 -> Mux/1
  Constant1/1 -> Discrete Notch/4
  Constant/1 -> Discrete Notch/3
  Demux/1 -> Discrete Notch/1
  Discrete Notch1/1 -> Mux/2
  Mux/1 -> dq_out/1
  Constant3/1 -> Discrete Notch1/4
  wnotch/1 -> Discrete Notch1/2, Discrete Notch/2
  Constant2/1 -> Discrete Notch1/3
  dq_in/1 -> Demux/1
  Demux/2 -> Discrete Notch1/1
